simulink model "Path_planner"  (R2017b)
settings: Solver=FixedStepDiscrete  StartTime=0.0  StopTime=20  FixedStep=dt  RelTol=1e-3
values from neighbouring files (symbols this model uses):
  dt = 0.1    [extendedKalmanFilter.m]    (also in matlab.mat; runV3.m; rungen.m; runpathfollower.m)
  pl = 4    [runpathfollower.m]    (also in runpathplanner.m = 10)
  pthetai = 45*pi/180    (= 0.785398163397)    [runpathfollower.m]    (also in runpathplanner.m)
  pxi = 2    [runpathfollower.m]    (also in runpathplanner.m = 0)
  pyi = 2    [runpathfollower.m]    (also in runpathplanner.m)
  velocity = 0.3    [runpathfollower.m]    (also in runpathplanner.m)
libraries: simulink x1
settings Model: Creator=nisha  LastModifiedBy=nisha

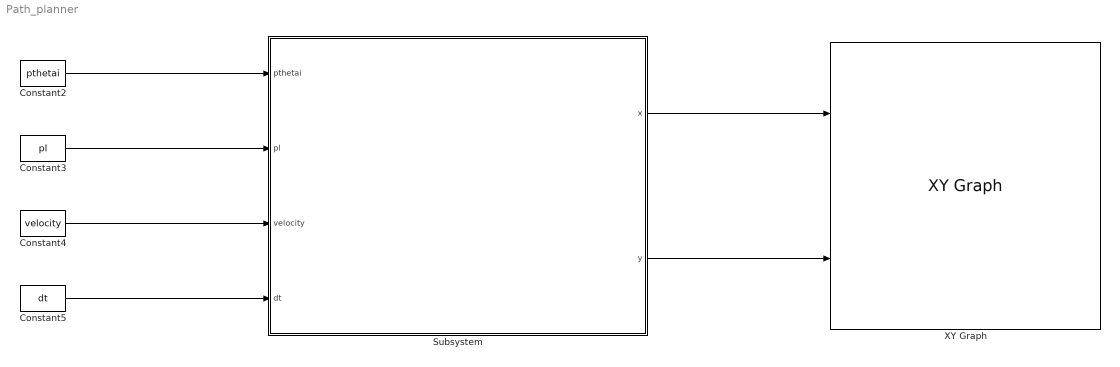
== system Path_planner ==
  Constant2 : Constant  Value=pthetai
  Constant3 : Constant  Value=pl
  Constant4 : Constant  Value=velocity
  Constant5 : Constant  Value=dt
  Subsystem : Subsystem
  XY Graph : simulink/Sinks/XY Graph  xmin=-1  xmax=9.5  ymin=-1  ymax=7  st=-1
  wires:
  Constant2/1 -> Subsystem/1(pthetai)
  Constant3/1 -> Subsystem/2(pl)
  Constant4/1 -> Subsystem/3(velocity)
  Subsystem/1(x) -> XY Graph/1
  Subsystem/2(y) -> XY Graph/2
  Constant5/1 -> Subsystem/4(dt)

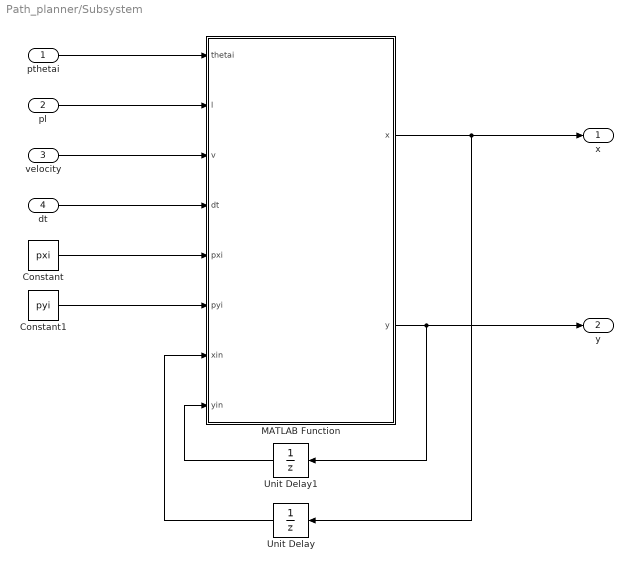
== system Path_planner/Subsystem ==
  pthetai : Inport
  pl : Inport  Port=2
  velocity : Inport  Port=3
  dt : Inport  Port=4
  Constant : Constant  Value=pxi
  Constant1 : Constant  Value=pyi
  MATLAB Function : MATLAB Function  TreatAsAtomicUnit=on
  Unit Delay : UnitDelay  InitialCondition=pxi  SampleTime=-1
  Unit Delay1 : UnitDelay  InitialCondition=pyi  SampleTime=-1
  x : Outport
  y : Outport  Port=2
  wires:
  pthetai/1 -> MATLAB Function/1(thetai)
  pl/1 -> MATLAB Function/2(l)
  velocity/1 -> MATLAB Function/3(v)
  MATLAB Function/1(x) -> Unit Delay/1, x/1
  MATLAB Function/2(y) -> Unit Delay1/1, y/1
  dt/1 -> MATLAB Function/4(dt)
  Unit Delay/1 -> MATLAB Function/7(xin)
  Unit Delay1/1 -> MATLAB Function/8(yin)
  Constant/1 -> MATLAB Function/5(pxi)
  Constant1/1 -> MATLAB Function/6(pyi)

== matlab function Path_planner/Subsystem/MATLAB Function ==
  data: x output; y output; thetai input; l input; v input; dt input; pxi input; pyi input; xin input; yin input
function [x,y] = fcn(thetai,l,v,dt,pxi,pyi,xin,yin)

dl=dt*v;
if abs(xin-pxi)<=(l-dl)*cos(thetai)
   x=xin+dl*cos(thetai); 
   y=yin+dl*sin(thetai);
else
    x=xin;
    y=yin;
end
end
